simulink model "ACC_OL"  (R2017b)
settings: Solver=VariableStepAuto  StartTime=0.0  StopTime=50  RelTol=1e-3
values from neighbouring files (symbols this model uses):
  a = 600    [InitCruiseControl.m]
  alpha = 20*pi/180    (= 0.349065850399)    [InitCruiseControl.m]
  b = 10    [InitCruiseControl.m]
  g = 9.81    [InitCruiseControl.m]    (also in nyquist1.m = gt(:,k))
  m = 1000    [InitCruiseControl.m]
settings Model: Creator=rizwanahmed  LastModifiedBy=rizwanahmed

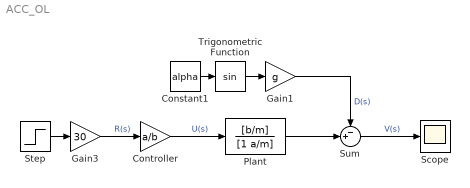
== system ACC_OL ==
  Constant1 : Constant  Value=alpha
  Controller : Gain  Gain=a/b
  Gain1 : Gain  Gain=g
  Gain3 : Gain  Gain=30
  Plant : TransferFcn  Numerator=[b/m]  Denominator=[1 a/m]
  Scope : Scope
  Step : Step  SampleTime=0
  Sum : Sum  Inputs=-+|
  Trigonometric Function : Trigonometry
  wires:
  Step/1 -> Gain3/1
  Constant1/1 -> Trigonometric Function/1
  Trigonometric Function/1 -> Gain1/1
  Gain3/1 -> Controller/1  "R(s)"
  Controller/1 -> Plant/1  "U(s)"
  Gain1/1 -> Sum/1  "D(s)"
  Plant/1 -> Sum/2
  Sum/1 -> Scope/1  "V(s)"
